simulink model "exam_2014"  (R2017a)
settings: Solver=VariableStepAuto  StartTime=0.0  StopTime=10.0  RelTol=1e-3
InitFcn:
  | clc
  | clear all
  | m=1
  | C_drag=1
  | A_front=1
  | Fmotor=1
  | p=1
settings Model: Creator=Martin  LastModifiedBy=Martin

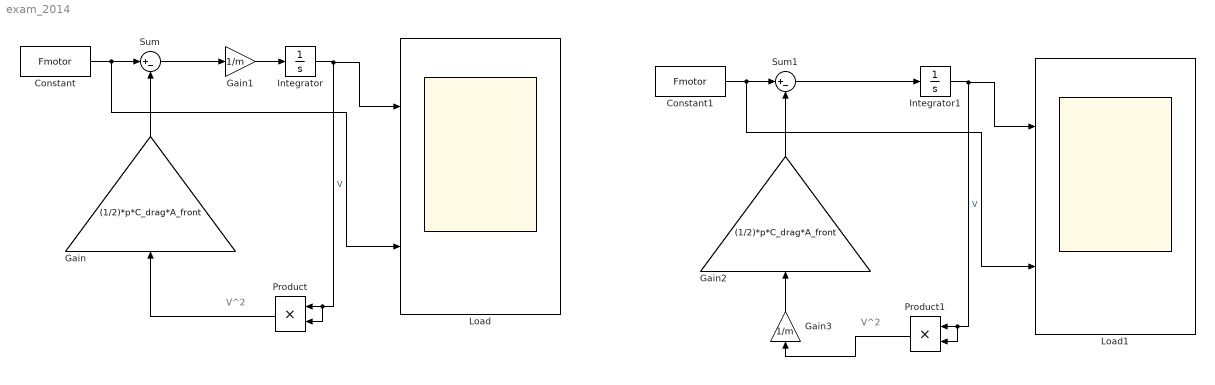
== system exam_2014 ==
  note: V^2
  note: V^2
  Constant : Constant  Value=Fmotor
  Constant1 : Constant  Value=Fmotor
  Gain : Gain  Gain=(1/2)*p*C_drag*A_front
  Gain1 : Gain  Gain=1/m
  Gain2 : Gain  Gain=(1/2)*p*C_drag*A_front
  Gain3 : Gain  Gain=1/m
  Integrator : Integrator
  Integrator1 : Integrator
  Load : Scope  NumInputPorts=2
  Load1 : Scope  NumInputPorts=2
  Product : Product
  Product1 : Product
  Sum : Sum  Inputs=|+-
  Sum1 : Sum  Inputs=|+-
  wires:
  Constant/1 -> Load/2, Sum/1
  Gain/1 -> Sum/2
  Product/1 -> Gain/1
  Sum/1 -> Gain1/1
  Gain1/1 -> Integrator/1
  Integrator/1 -> Load/1, Product/2, Product/1  "V"
  Integrator1/1 -> Product1/1, Product1/2, Load1/1  "V"
  Sum1/1 -> Integrator1/1
  Gain2/1 -> Sum1/2
  Constant1/1 -> Sum1/1, Load1/2
  Gain3/1 -> Gain2/1
  Product1/1 -> Gain3/1
